simulink model "Aircraft_WL1"  (R2017b)
settings: Solver=ode4  StartTime=0.0  StopTime=inf  FixedStep=Ts  RelTol=1e-3
libraries: aerolibfltsims x3, aerolibanimutils x1
settings Model: Creator=zht  LastModifiedBy=zht

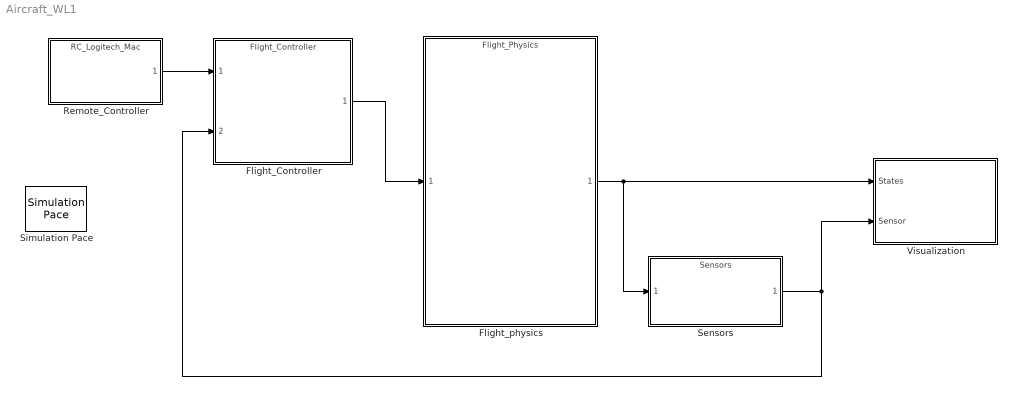
== system Aircraft_WL1 ==
  Flight_Controller : ModelReference  ModelNameDialog=Flight_Controller.slx  SimulationMode=Normal  ModelReferenceVersion=1.48
  Flight_physics : ModelReference  ModelNameDialog=Flight_Physics.slx  SimulationMode=Normal  ModelReferenceVersion=1.65
  Remote_Controller : ModelReference  ModelNameDialog=RC_Logitech_Mac.slx  SimulationMode=Normal  ModelReferenceVersion=1.7
  Sensors : ModelReference  ModelNameDialog=Sensors.slx  SimulationMode=Normal  ModelReferenceVersion=1.13
  Simulation Pace : aerolibanimutils/Simulation Pace  SimulationPace=1  SleepMode=MATLAB Thread  OutputPaceError=off  SampleTime=0.02
  Visualization : Subsystem
  wires:
  Flight_physics/1 -> Sensors/1, Visualization/1(States)
  Sensors/1 -> Visualization/2(Sensor), Flight_Controller/2
  Flight_Controller/1 -> Flight_physics/1
  Remote_Controller/1 -> Flight_Controller/1

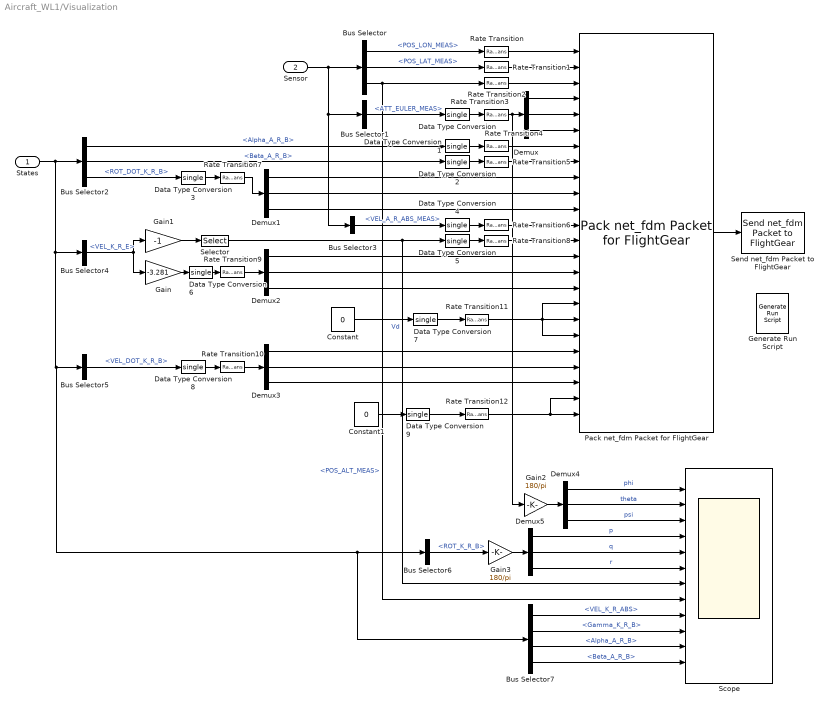
== system Aircraft_WL1/Visualization ==
  States : Inport  OutDataTypeStr=Bus: States_BUS
  Sensor : Inport  Port=2  OutDataTypeStr=Bus: Sensors_BUS
  Bus Selector : BusSelector  OutputSignals=POS_LON_MEAS,POS_LAT_MEAS,POS_ALT_MEAS
  Bus Selector1 : BusSelector  OutputSignals=ATT_EULER_MEAS
  Bus Selector2 : BusSelector  OutputSignals=Alpha_A_R_B,Beta_A_R_B,ROT_DOT_K_R_B
  Bus Selector3 : BusSelector  OutputSignals=VEL_A_R_ABS_MEAS
  Bus Selector4 : BusSelector  OutputSignals=VEL_K_R_E
  Bus Selector5 : BusSelector  OutputSignals=VEL_DOT_K_R_B
  Bus Selector6 : BusSelector  OutputSignals=ROT_K_R_B
  Bus Selector7 : BusSelector  OutputSignals=VEL_K_R_ABS,Gamma_K_R_B,Alpha_A_R_B,Beta_A_R_B
  Constant : Constant  Value=0
  Constant1 : Constant  Value=0
  Data Type Conversion{,1..9} (10 alike) : DataTypeConversion  OutDataTypeStr=single
  Demux{,1..5} (6 alike) : Demux  Outputs=3
  Gain : Gain  Gain=-3.281
  Gain1 : Gain  Gain=-1
  Gain2 : Gain  Gain=180/pi
  Gain3 : Gain  Gain=180/pi
  Generate Run Script : aerolibfltsims/Generate Run Script  OutputFileName=runfg.sh  FlightGearBaseDirectory=/Applications  GeometryModelName=c172p  DestinationPort=5502  OriginAddress=127.0.0.1  OriginPort=5505  LocalAddress=127.0.0.1  AirportId=KSFO  RunwayId=10L  InitialAltitude=7224  InitialHeading=113  OffsetDistance=4.72  OffsetAzimuth=0  GenerateFile=off  Architecture=Default  dataFlow=Send
  Pack net_fdm Packet for FlightGear : aerolibfltsims/Pack net_fdm Packet for FlightGear  FlightGearVersion=v2017.1  ShowPositionAttitudeInputs=on  ShowVelocityAccelerationInputs=on  ShowControlSurfacePositionInputs=off  ShowEngineFuelInputs=off  ShowLandingGearInputs=off  ShowEnvironmentInputs=off  SampleTime=0.02
      settings: SourceProductName=Aerospace Blockset  SourceProductBaseCode=AE
  Rate Transition{,1..12} (13 alike) : RateTransition  OutPortSampleTime=0.02
  Scope : Scope  NumInputPorts=12
  Selector : Selector  InputPortWidth=3  IndexOptions=Index vector (dialog)  Indices=[3]  OutputSizes=1
  Send net_fdm Packet to FlightGear : aerolibfltsims/Send net_fdm Packet to FlightGear  DestinationIpAddress=127.0.0.1  DestinationPort=5502  LocalIpPort=-1  varLen=off  SampleTime=0.02
      settings: SourceProductName=Aerospace Blockset  SourceProductBaseCode=AE
  wires:
  Pack net_fdm Packet for FlightGear/1 -> Send net_fdm Packet to FlightGear/1
  Sensor/1 -> Bus Selector/1, Bus Selector3/1, Bus Selector1/1
  Bus Selector/1 -> Rate Transition/1  "<POS_LON_MEAS>"
  Bus Selector/2 -> Rate Transition1/1  "<POS_LAT_MEAS>"
  Bus Selector/3 -> Scope/8, Rate Transition2/1  "<POS_ALT_MEAS>"
  Bus Selector1/1 -> Data Type Conversion/1  "<ATT_EULER_MEAS>"
  Demux/1 -> Pack net_fdm Packet for FlightGear/4
  Demux/2 -> Pack net_fdm Packet for FlightGear/5
  Demux/3 -> Pack net_fdm Packet for FlightGear/6
  Bus Selector2/1 -> Data Type Conversion1/1  "<Alpha_A_R_B>"
  Bus Selector2/2 -> Data Type Conversion2/1  "<Beta_A_R_B>"
  Bus Selector2/3 -> Data Type Conversion3/1  "<ROT_DOT_K_R_B>"
  Demux1/2 -> Pack net_fdm Packet for FlightGear/10
  Demux1/3 -> Pack net_fdm Packet for FlightGear/11
  Bus Selector3/1 -> Data Type Conversion4/1  "<VEL_A_R_ABS_MEAS>"
  States/1 -> Bus Selector7/1, Bus Selector6/1, Bus Selector5/1, Bus Selector4/1, Bus Selector2/1
  Bus Selector4/1 -> Gain/1, Gain1/1  "<VEL_K_R_E>"
  Selector/1 -> Scope/7, Data Type Conversion5/1  "Vd"
  Demux2/1 -> Pack net_fdm Packet for FlightGear/14
  Demux2/2 -> Pack net_fdm Packet for FlightGear/15
  Demux2/3 -> Pack net_fdm Packet for FlightGear/16
  Gain/1 -> Data Type Conversion6/1
  Constant/1 -> Data Type Conversion7/1
  Bus Selector5/1 -> Data Type Conversion8/1  "<VEL_DOT_K_R_B>"
  Demux3/1 -> Pack net_fdm Packet for FlightGear/20
  Demux3/2 -> Pack net_fdm Packet for FlightGear/21
  Demux3/3 -> Pack net_fdm Packet for FlightGear/22
  Rate Transition/1 -> Pack net_fdm Packet for FlightGear/1
  Rate Transition1/1 -> Pack net_fdm Packet for FlightGear/2
  Rate Transition2/1 -> Pack net_fdm Packet for FlightGear/3
  Rate Transition3/1 -> Gain2/1, Demux/1
  Rate Transition4/1 -> Pack net_fdm Packet for FlightGear/7
  Rate Transition5/1 -> Pack net_fdm Packet for FlightGear/8
  Demux1/1 -> Pack net_fdm Packet for FlightGear/9
  Rate Transition7/1 -> Demux1/1
  Rate Transition9/1 -> Demux2/1
  Rate Transition10/1 -> Demux3/1
  Rate Transition11/1 -> Pack net_fdm Packet for FlightGear/19, Pack net_fdm Packet for FlightGear/17, Pack net_fdm Packet for FlightGear/18
  Rate Transition12/1 -> Pack net_fdm Packet for FlightGear/24, Pack net_fdm Packet for FlightGear/23
  Constant1/1 -> Data Type Conversion9/1
  Data Type Conversion/1 -> Rate Transition3/1
  Data Type Conversion1/1 -> Rate Transition4/1
  Data Type Conversion2/1 -> Rate Transition5/1
  Data Type Conversion3/1 -> Rate Transition7/1
  Data Type Conversion4/1 -> Rate Transition6/1
  Data Type Conversion5/1 -> Rate Transition8/1
  Data Type Conversion6/1 -> Rate Transition9/1
  Data Type Conversion7/1 -> Rate Transition11/1
  Data Type Conversion8/1 -> Rate Transition10/1
  Data Type Conversion9/1 -> Rate Transition12/1
  Rate Transition6/1 -> Pack net_fdm Packet for FlightGear/12
  Rate Transition8/1 -> Pack net_fdm Packet for FlightGear/13
  Gain1/1 -> Selector/1
  Demux4/1 -> Scope/1  "phi"
  Demux4/2 -> Scope/2  "theta"
  Demux4/3 -> Scope/3  "psi"
  Gain2/1 -> Demux4/1
  Bus Selector6/1 -> Gain3/1  "<ROT_K_R_B>"
  Gain3/1 -> Demux5/1
  Demux5/2 -> Scope/5  "q"
  Demux5/1 -> Scope/4  "p"
  Demux5/3 -> Scope/6  "r"
  Bus Selector7/4 -> Scope/12  "<Beta_A_R_B>"
  Bus Selector7/1 -> Scope/9  "<VEL_K_R_ABS>"
  Bus Selector7/2 -> Scope/10  "<Gamma_K_R_B>"
  Bus Selector7/3 -> Scope/11  "<Alpha_A_R_B>"
